simulink library "CoCoSTLib_R2015b"  (R2015b)
settings: Solver=ode45  StartTime=0.0  StopTime=10.0  RelTol=1e-3
libraries: CoCoSTLib_R2015b x31
settings Model: Creator=balsi  LastModifiedBy=xiayu
settings DataIOCC: SaveFormat=Array
settings DebuggingCC: AllowSymbolicDim=on
settings HardwareCC: ProdBitPerPointer=32  ProdLargestAtomicFloat=None  ProdIntDivRoundTo=Undefined  ProdEndianess=Unspecified  ProdWordSize=32  ProdHWDeviceType=32-bit Generic
settings ConfigComp: CovHtmlReporting=off  CovModelRefEnable=Off

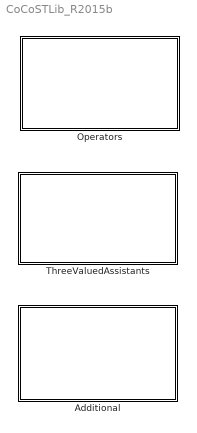
== system CoCoSTLib_R2015b ==
  Additional : Subsystem
      mask Display: disp('Additional')
  Operators : Subsystem
      mask Display: disp("Operators")
  ThreeValuedAssistants : Subsystem
      mask Display: disp("Enablers - Three Valued")

== system CoCoSTLib_R2015b/Additional ==
  note: Additional
  And_nested : Subsystem
  DelaySTL : Subsystem
  DelayedTimeWindow : Subsystem
  TimeWindow : Subsystem

== system CoCoSTLib_R2015b/Operators ==
  Operators_3V : Subsystem
      mask Display: disp("Operators Three-valued Logic")
  Operators_LF : Subsystem
      mask Display: disp('Operators LogicT')
  Operators_LT : Subsystem
      mask Display: disp('Operators LogicF')

== system CoCoSTLib_R2015b/ThreeValuedAssistants ==
  note: In order to save memory, values can be encoded in two digits.
      | For example:
      | 	True: [1, 1]
      |        False: [ 0, 0]
      |        Unknown: [1, 0]
  note: 3V assistants
  note: 3V assignments
  AND_3V : Subsystem
  False_3V : Subsystem
      mask Display: disp("F_3V")
  "Interpreter " : Subsystem
  NOT_3V : Subsystem
  OR_3V : Subsystem
  True_3V : Subsystem
      mask Display: disp("T_3V")
  Unknown_3V : Subsystem
      mask Display: disp("U_3V")

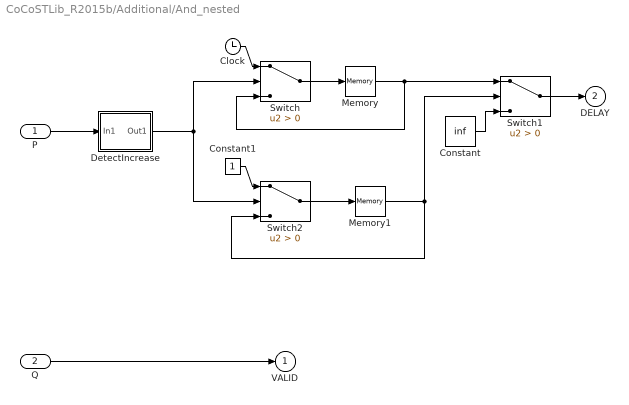
== system CoCoSTLib_R2015b/Additional/And_nested ==
  P : Inport
  Q : Inport  Port=2
  Clock : Clock
  Constant : Constant  Value=inf
  Constant1 : Constant
  DetectIncrease : Subsystem
  Memory : Memory
  Memory1 : Memory
  Switch : Switch  Criteria=u2 > Threshold
  Switch1 : Switch  Criteria=u2 > Threshold
  Switch2 : Switch  Criteria=u2 > Threshold
  VALID : Outport
  DELAY : Outport  Port=2
  wires:
  Q/1 -> VALID/1
  Memory/1 -> Switch1/1, Switch/3
  Memory1/1 -> Switch1/2, Switch2/3
  Switch/1 -> Memory/1
  Switch1/1 -> DELAY/1
  Constant/1 -> Switch1/3
  Switch2/1 -> Memory1/1
  Constant1/1 -> Switch2/1
  Clock/1 -> Switch/1
  DetectIncrease/1(Out1) -> Switch2/2, Switch/2
  P/1 -> DetectIncrease/1(In1)

== system CoCoSTLib_R2015b/Additional/DelaySTL ==
  IN : Inport
  Clock : Clock
  Constant : Constant  Value=inf
  Constant1 : Constant
  DetectIncrease : Subsystem
  Memory : Memory
  Memory1 : Memory
  Switch : Switch  Criteria=u2 > Threshold
  Switch1 : Switch  Criteria=u2 > Threshold
  Switch2 : Switch  Criteria=u2 > Threshold
  OUT : Outport
  wires:
  Clock/1 -> Switch/1
  Constant1/1 -> Switch2/1
  Memory1/1 -> Switch1/2, Switch2/3
  Switch/1 -> Memory/1
  Switch1/1 -> OUT/1
  Switch2/1 -> Memory1/1
  DetectIncrease/1(Y) -> Switch/2, Switch2/2
  IN/1 -> DetectIncrease/1(U)
  Memory/1 -> Switch1/1, Switch/3
  Constant/1 -> Switch1/3

== system CoCoSTLib_R2015b/Additional/DelayedTimeWindow ==
  T_Start : Inport
  T_End : Inport  Port=2
  DELAY : Inport  Port=3
  AND1 : Logic  AllPortsSameDT=off  OutDataTypeStr=boolean
  CLOCK : Clock
  DELAY_SUB : Sum  Inputs=+-
  REL1 : RelationalOperator  Operator=<=  OutDataTypeStr=boolean
  REL2 : RelationalOperator  Operator=<=  OutDataTypeStr=boolean
  OUT : Outport
  wires:
  REL1/1 -> AND1/1
  CLOCK/1 -> DELAY_SUB/1
  REL2/1 -> AND1/2
  T_Start/1 -> REL1/1
  DELAY_SUB/1 -> REL1/2, REL2/1
  AND1/1 -> OUT/1
  DELAY/1 -> DELAY_SUB/2
  T_End/1 -> REL2/2

== system CoCoSTLib_R2015b/Additional/TimeWindow ==
  T_Start : Inport
  T_End : Inport  Port=2
  AND : Logic  AllPortsSameDT=off  OutDataTypeStr=boolean
  CLOCK : Clock
  REL1 : RelationalOperator  Operator=<=  OutDataTypeStr=boolean
  REL2 : RelationalOperator  Operator=<=  OutDataTypeStr=boolean
  OUT : Outport
  wires:
  CLOCK/1 -> REL1/2, REL2/1
  T_End/1 -> REL2/2
  REL1/1 -> AND/1
  REL2/1 -> AND/2
  AND/1 -> OUT/1
  T_Start/1 -> REL1/1

== system CoCoSTLib_R2015b/Operators/Operators_3V ==
  Always_3V : Subsystem
  Eventually_3V : Subsystem
  Until_3V : Subsystem

== system CoCoSTLib_R2015b/Operators/Operators_LF ==
  Always_LF : Subsystem
  Eventually_LF : Subsystem
      mask Display: disp('Eventuall LogicF')
  Eventually_LFbis : Subsystem  Commented=on
  Until_LF : Subsystem

== system CoCoSTLib_R2015b/Operators/Operators_LT ==
  "Always_LT " : Subsystem
  Always_LT_timewindows : Subsystem  Commented=on
  Always_LTbis : Subsystem  Commented=on
  "Eventually_LT " : Subsystem
  Eventually_LT bis : Subsystem  Commented=on
  Eventually_T : Subsystem  Commented=on
  Until_LT : Subsystem

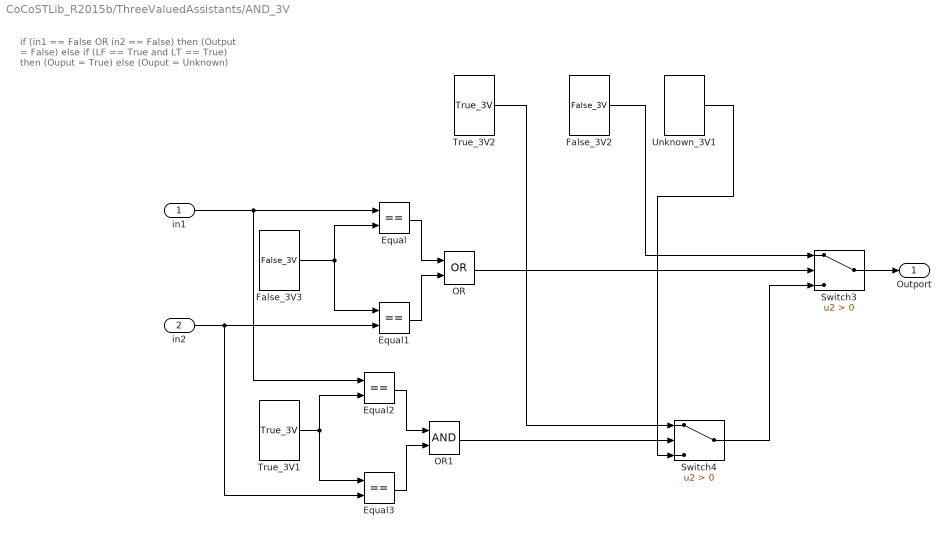
== system CoCoSTLib_R2015b/ThreeValuedAssistants/AND_3V ==
  note: if (in1 == False OR in2 == False)
      | then (Output = False)
      | else if (LF == True and LT == True)
      | then (Ouput = True)
      | else (Ouput = Unknown)
  "in1 " : Inport
  in2 : Inport  Port=2
  Equal{,1..3} (4 alike) : RelationalOperator  Operator===  OutDataTypeStr=boolean
  False_3V2 : CoCoSTLib_R2015b/ThreeValuedAssistants/False_3V  SystemSampleTime=-1  Latency=0  AutoFrameSizeCalculation=off
  False_3V3 : CoCoSTLib_R2015b/ThreeValuedAssistants/False_3V  SystemSampleTime=-1  Latency=0  AutoFrameSizeCalculation=off
  OR : Logic  Operator=OR  AllPortsSameDT=off  OutDataTypeStr=boolean
  OR1 : Logic  AllPortsSameDT=off  OutDataTypeStr=boolean
  Switch3 : Switch  Criteria=u2 > Threshold
  Switch4 : Switch  Criteria=u2 > Threshold
  True_3V1 : CoCoSTLib_R2015b/ThreeValuedAssistants/True_3V  SystemSampleTime=-1  Latency=0  AutoFrameSizeCalculation=off
  True_3V2 : CoCoSTLib_R2015b/ThreeValuedAssistants/True_3V  SystemSampleTime=-1  Latency=0  AutoFrameSizeCalculation=off
  Unknown_3V1 : CoCoSTLib_R2015b/ThreeValuedAssistants/Unknown_3V  SystemSampleTime=-1  Latency=0  AutoFrameSizeCalculation=off
  Outport : Outport
  wires:
  False_3V3/1 -> Equal/2, Equal1/1
  Equal/1 -> OR/1
  Equal1/1 -> OR/2
  OR/1 -> Switch3/2
  Switch3/1 -> Outport/1
  Equal2/1 -> OR1/1
  Equal3/1 -> OR1/2
  OR1/1 -> Switch4/2
  "in1 "/1 -> Equal2/1, Equal/1
  True_3V1/1 -> Equal2/2, Equal3/1
  in2/1 -> Equal1/2, Equal3/2
  True_3V2/1 -> Switch4/1
  Switch4/1 -> Switch3/3
  False_3V2/1 -> Switch3/1
  Unknown_3V1/1 -> Switch4/3

== system CoCoSTLib_R2015b/ThreeValuedAssistants/False_3V ==
  Constant1 : Constant  Value=0
  Out1 : Outport
  wires:
  Constant1/1 -> Out1/1

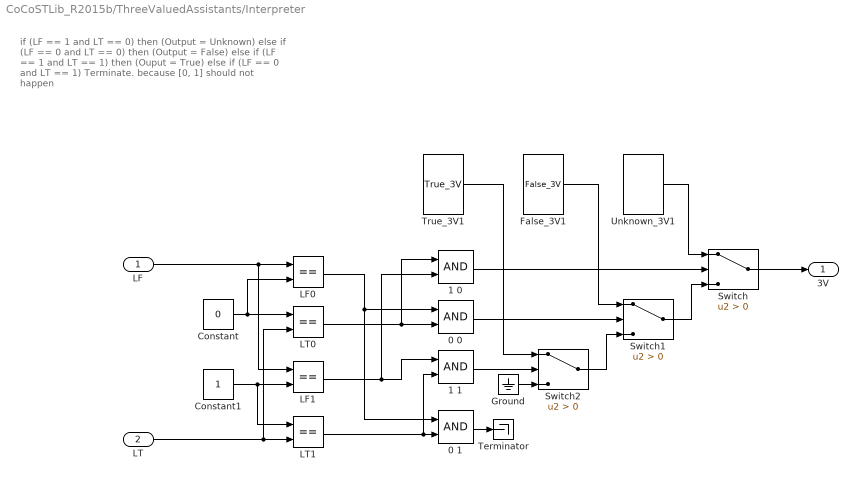
== system CoCoSTLib_R2015b/ThreeValuedAssistants/Interpreter  ==
  note: if (LF == 1 and LT == 0)
      | then (Output = Unknown)
      | else if (LF == 0 and LT == 0)
      | then (Output = False)
      | else if (LF == 1 and LT == 1)
      | then (Ouput = True)
      | else if (LF == 0 and LT == 1)
      | Terminate.
      | because [0, 1] should not happen
  LF : Inport
  LT : Inport  Port=2
  0 0 : Logic  AllPortsSameDT=off  OutDataTypeStr=boolean
  0 1 : Logic  AllPortsSameDT=off  OutDataTypeStr=boolean
  1 0 : Logic  AllPortsSameDT=off  OutDataTypeStr=boolean
  1 1 : Logic  AllPortsSameDT=off  OutDataTypeStr=boolean
  Constant : Constant  Value=0
  Constant1 : Constant
  False_3V1 : CoCoSTLib_R2015b/ThreeValuedAssistants/False_3V  SystemSampleTime=-1  Latency=0  AutoFrameSizeCalculation=off
  Ground : Ground
  LF0 : RelationalOperator  Operator===  OutDataTypeStr=boolean
  LF1 : RelationalOperator  Operator===  OutDataTypeStr=boolean
  "LT0 " : RelationalOperator  Operator===  OutDataTypeStr=boolean
  "LT1 " : RelationalOperator  Operator===  OutDataTypeStr=boolean
  Switch : Switch  Criteria=u2 > Threshold
  Switch1 : Switch  Criteria=u2 > Threshold
  Switch2 : Switch  Criteria=u2 > Threshold
  Terminator : Terminator
  True_3V1 : CoCoSTLib_R2015b/ThreeValuedAssistants/True_3V  SystemSampleTime=-1  Latency=0  AutoFrameSizeCalculation=off
  Unknown_3V1 : CoCoSTLib_R2015b/ThreeValuedAssistants/Unknown_3V  SystemSampleTime=-1  Latency=0  AutoFrameSizeCalculation=off
  3V : Outport
  wires:
  Constant/1 -> "LT0 "/1, LF0/2
  1 0/1 -> Switch/2
  Switch/1 -> 3V/1
  Constant1/1 -> LF1/2, "LT1 "/1
  LF1/1 -> 1 1/1, 1 0/2
  0 0/1 -> Switch1/2
  Switch1/1 -> Switch/3
  "LT0 "/1 -> 0 0/2, 1 0/1
  LF0/1 -> 0 1/1, 0 0/1
  "LT1 "/1 -> 1 1/2, 0 1/2
  1 1/1 -> Switch2/2
  Switch2/1 -> Switch1/3
  0 1/1 -> Terminator/1
  Ground/1 -> Switch2/3
  Unknown_3V1/1 -> Switch/1
  True_3V1/1 -> Switch2/1
  False_3V1/1 -> Switch1/1
  LF/1 -> LF1/1, LF0/1
  LT/1 -> "LT0 "/2, "LT1 "/2

== system CoCoSTLib_R2015b/ThreeValuedAssistants/NOT_3V ==
  note: if (in == True)
      | then (Output = False)
      | else if (in == False)
      | then (Ouput = True)
      | else (Ouput = Unknown)
  "Input " : Inport
  Equal : RelationalOperator  Operator===  OutDataTypeStr=boolean
  Equal2 : RelationalOperator  Operator===  OutDataTypeStr=boolean
  False_3V1 : CoCoSTLib_R2015b/ThreeValuedAssistants/False_3V  SystemSampleTime=-1  Latency=0  AutoFrameSizeCalculation=off
  False_3V2 : CoCoSTLib_R2015b/ThreeValuedAssistants/False_3V  SystemSampleTime=-1  Latency=0  AutoFrameSizeCalculation=off
  Switch3 : Switch  Criteria=u2 > Threshold
  Switch4 : Switch  Criteria=u2 > Threshold
  True_3V2 : CoCoSTLib_R2015b/ThreeValuedAssistants/True_3V  SystemSampleTime=-1  Latency=0  AutoFrameSizeCalculation=off
  True_3V3 : CoCoSTLib_R2015b/ThreeValuedAssistants/True_3V  SystemSampleTime=-1  Latency=0  AutoFrameSizeCalculation=off
  Unknown_3V1 : CoCoSTLib_R2015b/ThreeValuedAssistants/Unknown_3V  SystemSampleTime=-1  Latency=0  AutoFrameSizeCalculation=off
  Outport : Outport
  wires:
  Switch3/1 -> Outport/1
  False_3V1/1 -> Equal2/2
  Equal/1 -> Switch3/2
  "Input "/1 -> Equal2/1, Equal/1
  False_3V2/1 -> Switch3/1
  True_3V3/1 -> Equal/2
  Unknown_3V1/1 -> Switch4/3
  Switch4/1 -> Switch3/3
  True_3V2/1 -> Switch4/1
  Equal2/1 -> Switch4/2

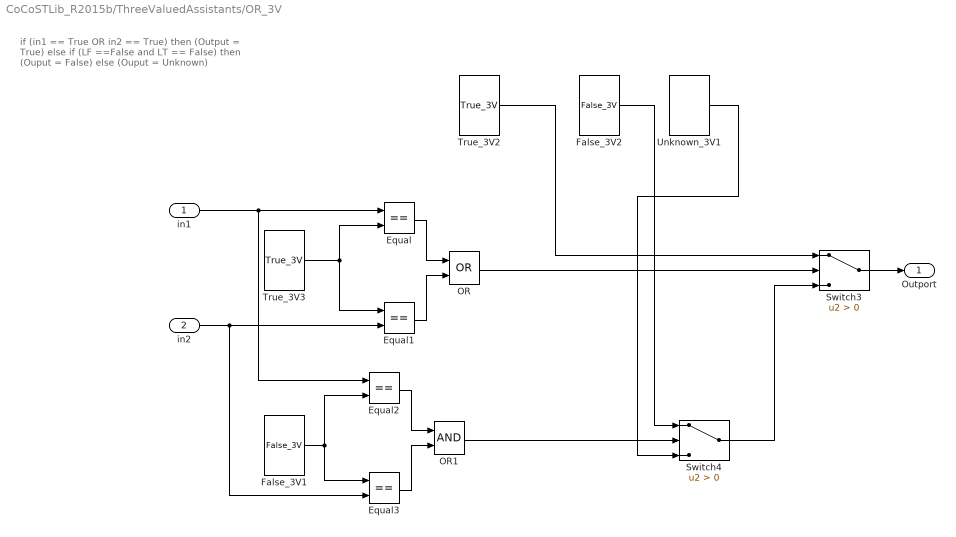
== system CoCoSTLib_R2015b/ThreeValuedAssistants/OR_3V ==
  note: if (in1 == True OR in2 == True)
      | then (Output = True)
      | else if (LF ==False and LT == False)
      | then (Ouput = False)
      | else (Ouput = Unknown)
  "in1 " : Inport
  in2 : Inport  Port=2
  Equal{,1..3} (4 alike) : RelationalOperator  Operator===  OutDataTypeStr=boolean
  False_3V1 : CoCoSTLib_R2015b/ThreeValuedAssistants/False_3V  SystemSampleTime=-1  Latency=0  AutoFrameSizeCalculation=off
  False_3V2 : CoCoSTLib_R2015b/ThreeValuedAssistants/False_3V  SystemSampleTime=-1  Latency=0  AutoFrameSizeCalculation=off
  OR : Logic  Operator=OR  AllPortsSameDT=off  OutDataTypeStr=boolean
  OR1 : Logic  AllPortsSameDT=off  OutDataTypeStr=boolean
  Switch3 : Switch  Criteria=u2 > Threshold
  Switch4 : Switch  Criteria=u2 > Threshold
  True_3V2 : CoCoSTLib_R2015b/ThreeValuedAssistants/True_3V  SystemSampleTime=-1  Latency=0  AutoFrameSizeCalculation=off
  True_3V3 : CoCoSTLib_R2015b/ThreeValuedAssistants/True_3V  SystemSampleTime=-1  Latency=0  AutoFrameSizeCalculation=off
  Unknown_3V1 : CoCoSTLib_R2015b/ThreeValuedAssistants/Unknown_3V  SystemSampleTime=-1  Latency=0  AutoFrameSizeCalculation=off
  Outport : Outport
  wires:
  True_3V3/1 -> Equal/2, Equal1/1
  Equal/1 -> OR/1
  Equal1/1 -> OR/2
  OR/1 -> Switch3/2
  Unknown_3V1/1 -> Switch4/3
  Switch3/1 -> Outport/1
  Equal2/1 -> OR1/1
  Equal3/1 -> OR1/2
  OR1/1 -> Switch4/2
  "in1 "/1 -> Equal2/1, Equal/1
  False_3V1/1 -> Equal2/2, Equal3/1
  in2/1 -> Equal1/2, Equal3/2
  False_3V2/1 -> Switch4/1
  Switch4/1 -> Switch3/3
  True_3V2/1 -> Switch3/1

== system CoCoSTLib_R2015b/ThreeValuedAssistants/True_3V ==
  Constant : Constant
  Out1 : Outport
  wires:
  Constant/1 -> Out1/1

== system CoCoSTLib_R2015b/ThreeValuedAssistants/Unknown_3V ==
  Constant2 : Constant  Value=-1
  Out1 : Outport
  wires:
  Constant2/1 -> Out1/1

== system CoCoSTLib_R2015b/Additional/And_nested/DetectIncrease ==
  note: U(k)
  note: Edge
  In1 : Inport
  FixPt Relational Operator : RelationalOperator  Operator=>  OutDataTypeStr=boolean  ZeroCross=off
  Memory : Memory
  Out1 : Outport
  wires:
  In1/1 -> Memory/1, FixPt Relational Operator/1
  Memory/1 -> FixPt Relational Operator/2  "U(k-1)"
  FixPt Relational Operator/1 -> Out1/1

== system CoCoSTLib_R2015b/Additional/DelaySTL/DetectIncrease ==
  note: U(k)
  note: Edge
  U : Inport
  FixPt Relational Operator : RelationalOperator  Operator=>  OutDataTypeStr=boolean  ZeroCross=off
  Memory : Memory
  Y : Outport  InitialOutput=0
  wires:
  Memory/1 -> FixPt Relational Operator/2  "U(k-1)"
  FixPt Relational Operator/1 -> Y/1
  U/1 -> Memory/1, FixPt Relational Operator/1

== system CoCoSTLib_R2015b/Operators/Operators_3V/Always_3V ==
  "T_start " : Inport
  "T_end " : Inport  Port=2
  P : Inport  Port=3
  Always LF : CoCoSTLib_R2015b/Operators/Operators_LF/Always_LF  SystemSampleTime=-1  Latency=0  AutoFrameSizeCalculation=off
  "Always LT " : CoCoSTLib_R2015b/Operators/Operators_LT/Always_LT   SystemSampleTime=-1  Latency=0  AutoFrameSizeCalculation=off
  "Interpreter " : CoCoSTLib_R2015b/ThreeValuedAssistants/Interpreter   SystemSampleTime=-1  Latency=0  AutoFrameSizeCalculation=off
  3V : Outport
  wires:
  "T_end "/1 -> "Always LT "/2, Always LF/2
  Always LF/1 -> "Interpreter "/1
  "Interpreter "/1 -> 3V/1
  "T_start "/1 -> Always LF/1, "Always LT "/1
  P/1 -> Always LF/3, "Always LT "/3
  "Always LT "/1 -> "Interpreter "/2

== system CoCoSTLib_R2015b/Operators/Operators_3V/Eventually_3V ==
  "T_start " : Inport
  "T_end " : Inport  Port=2
  P : Inport  Port=3
  Eventually LF : CoCoSTLib_R2015b/Operators/Operators_LF/Eventually_LF  SystemSampleTime=-1  Latency=0  AutoFrameSizeCalculation=off
  "Eventually LT " : CoCoSTLib_R2015b/Operators/Operators_LT/Eventually_LT   SystemSampleTime=-1  Latency=0  AutoFrameSizeCalculation=off
  "Interpreter " : CoCoSTLib_R2015b/ThreeValuedAssistants/Interpreter   SystemSampleTime=-1  Latency=0  AutoFrameSizeCalculation=off
  3V : Outport
  wires:
  Eventually LF/1 -> "Interpreter "/1
  "Eventually LT "/1 -> "Interpreter "/2
  P/1 -> "Eventually LT "/3, Eventually LF/3
  "T_end "/1 -> "Eventually LT "/2, Eventually LF/2
  "Interpreter "/1 -> 3V/1
  "T_start "/1 -> "Eventually LT "/1, Eventually LF/1

== system CoCoSTLib_R2015b/Operators/Operators_3V/Until_3V ==
  "T_start " : Inport
  "T_end " : Inport  Port=2
  P : Inport  Port=3
  "Q " : Inport  Port=4
  "Interpreter " : CoCoSTLib_R2015b/ThreeValuedAssistants/Interpreter   SystemSampleTime=-1  Latency=0  AutoFrameSizeCalculation=off
  Until LF : CoCoSTLib_R2015b/Operators/Operators_LF/Until_LF  SystemSampleTime=-1  Latency=0  AutoFrameSizeCalculation=off
  Until LT : CoCoSTLib_R2015b/Operators/Operators_LT/Until_LT  SystemSampleTime=-1  Latency=0  AutoFrameSizeCalculation=off
  3V : Outport
  wires:
  "T_end "/1 -> Until LF/2, Until LT/2
  "T_start "/1 -> Until LT/1, Until LF/1
  "Q "/1 -> Until LF/4, Until LT/4
  P/1 -> Until LF/3, Until LT/3
  "Interpreter "/1 -> 3V/1
  Until LT/1 -> "Interpreter "/2
  Until LF/1 -> "Interpreter "/1

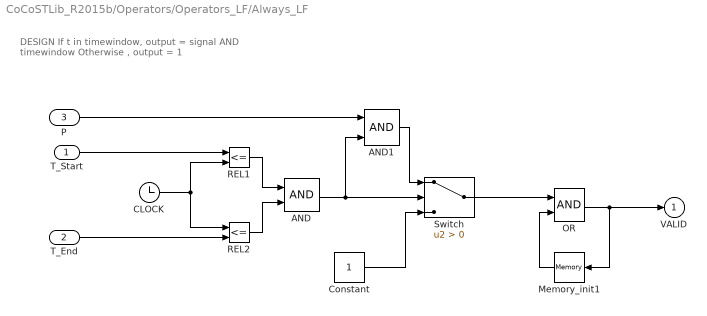
== system CoCoSTLib_R2015b/Operators/Operators_LF/Always_LF ==
  note: DESIGN
      | If t in timewindow, output = signal AND timewindow
      | Otherwise , output = 1
  T_Start : Inport
  T_End : Inport  Port=2
  P : Inport  Port=3
  AND : Logic  AllPortsSameDT=off  OutDataTypeStr=boolean
  AND1 : Logic  AllPortsSameDT=off  OutDataTypeStr=boolean
  CLOCK : Clock
  Constant : Constant
  Memory_init1 : Memory  X0=1
  OR : Logic  AllPortsSameDT=off  OutDataTypeStr=boolean
  REL1 : RelationalOperator  Operator=<=  OutDataTypeStr=boolean
  REL2 : RelationalOperator  Operator=<=  OutDataTypeStr=boolean
  Switch : Switch  Criteria=u2 > Threshold
  VALID : Outport
  wires:
  AND1/1 -> Switch/1
  CLOCK/1 -> REL2/1, REL1/2
  Memory_init1/1 -> OR/2
  Switch/1 -> OR/1
  T_End/1 -> REL2/2
  OR/1 -> VALID/1, Memory_init1/1
  T_Start/1 -> REL1/1
  Constant/1 -> Switch/3
  REL1/1 -> AND/1
  REL2/1 -> AND/2
  AND/1 -> AND1/2, Switch/2
  P/1 -> AND1/1

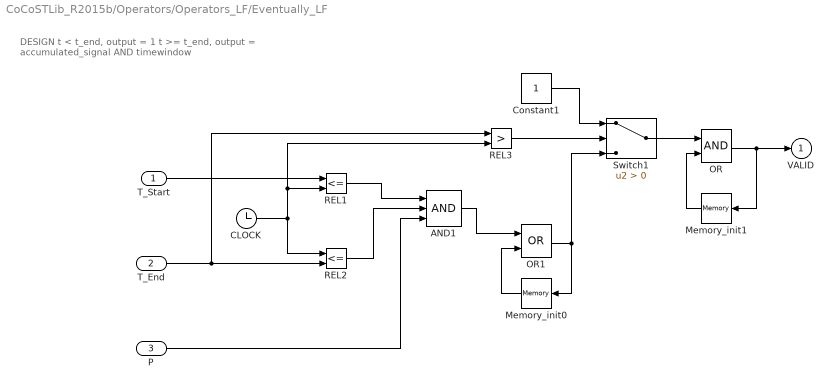
== system CoCoSTLib_R2015b/Operators/Operators_LF/Eventually_LF ==
  note: DESIGN
      | t < t_end, output = 1
      | t >= t_end, output = accumulated_signal AND timewindow
  T_Start : Inport
  T_End : Inport  Port=2
  P : Inport  Port=3
  AND1 : Logic  Inputs=3  AllPortsSameDT=off  OutDataTypeStr=boolean
  CLOCK : Clock
  Constant1 : Constant
  "Memory_init0 " : Memory
  Memory_init1 : Memory  X0=1
  OR : Logic  AllPortsSameDT=off  OutDataTypeStr=boolean
  OR1 : Logic  Operator=OR  AllPortsSameDT=off  OutDataTypeStr=boolean
  REL1 : RelationalOperator  Operator=<=  OutDataTypeStr=boolean
  REL2 : RelationalOperator  Operator=<=  OutDataTypeStr=boolean
  REL3 : RelationalOperator  Operator=>  OutDataTypeStr=boolean
  Switch1 : Switch  Criteria=u2 > Threshold
  VALID : Outport
  wires:
  T_End/1 -> REL3/1, REL2/2
  AND1/1 -> OR1/1
  REL1/1 -> AND1/1
  P/1 -> AND1/3
  CLOCK/1 -> REL3/2, REL1/2, REL2/1
  T_Start/1 -> REL1/1
  "Memory_init0 "/1 -> OR1/2
  OR1/1 -> "Memory_init0 "/1, Switch1/3
  Constant1/1 -> Switch1/1
  REL2/1 -> AND1/2
  REL3/1 -> Switch1/2
  Memory_init1/1 -> OR/2
  OR/1 -> VALID/1, Memory_init1/1
  Switch1/1 -> OR/1

== system CoCoSTLib_R2015b/Operators/Operators_LF/Eventually_LFbis ==
  note: DESIGN
      | t < t_end, output = 1
      | t >= t_end, output = accumulated_signal AND timewindow
  T_Start : Inport
  T_End : Inport  Port=2
  P : Inport  Port=3
  AND2 : Logic  AllPortsSameDT=off  OutDataTypeStr=boolean
  Always LF : CoCoSTLib_R2015b/Operators_LF/Always_LF  SystemSampleTime=-1  Latency=0  AutoFrameSizeCalculation=off
  CLOCK1 : Clock
  Memory_init1 : Memory  X0=1
  NOT : Logic  Operator=NOT  IconShape=distinctive  AllPortsSameDT=off  OutDataTypeStr=boolean
  NOT1 : Logic  Operator=NOT  IconShape=distinctive  AllPortsSameDT=off  OutDataTypeStr=boolean
  OR : Logic  AllPortsSameDT=off  OutDataTypeStr=boolean
  REL4 : RelationalOperator  Operator=<=  OutDataTypeStr=boolean
  VALID : Outport
  wires:
  T_Start/1 -> Always LF/1
  T_End/1 -> Always LF/2, REL4/1
  P/1 -> NOT/1
  NOT/1 -> Always LF/3
  CLOCK1/1 -> REL4/2
  Always LF/1 -> AND2/1
  REL4/1 -> AND2/2
  AND2/1 -> NOT1/1
  Memory_init1/1 -> OR/2
  NOT1/1 -> OR/1
  OR/1 -> VALID/1, Memory_init1/1

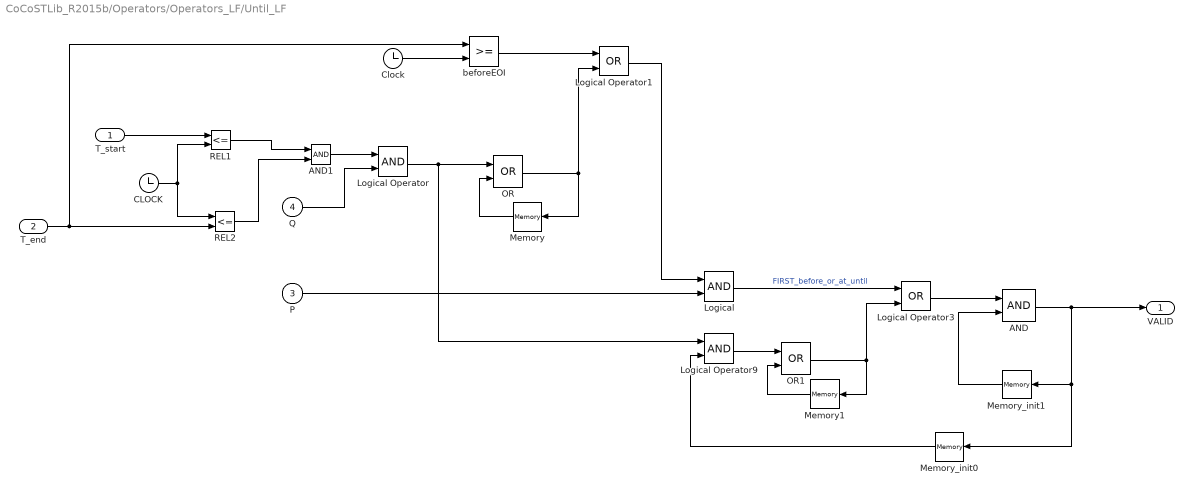
== system CoCoSTLib_R2015b/Operators/Operators_LF/Until_LF ==
  "T_start " : Inport
  T_end : Inport  Port=2
  P : Inport  Port=3
  Q : Inport  Port=4
  AND : Logic  AllPortsSameDT=off  OutDataTypeStr=boolean
  AND1 : Logic  AllPortsSameDT=off  OutDataTypeStr=boolean
  CLOCK : Clock
  Clock : Clock
  "Logical " : Logic  AllPortsSameDT=off  OutDataTypeStr=boolean
  Logical Operator : Logic  AllPortsSameDT=off  OutDataTypeStr=boolean
  Logical Operator1 : Logic  Operator=OR  AllPortsSameDT=off  OutDataTypeStr=boolean
  Logical Operator3 : Logic  Operator=OR  AllPortsSameDT=off  OutDataTypeStr=boolean
  Logical Operator9 : Logic  AllPortsSameDT=off  OutDataTypeStr=boolean
  Memory : Memory
  Memory1 : Memory
  "Memory_init0 " : Memory
  Memory_init1 : Memory  X0=1
  OR : Logic  Operator=OR  AllPortsSameDT=off  OutDataTypeStr=boolean
  OR1 : Logic  Operator=OR  AllPortsSameDT=off  OutDataTypeStr=boolean
  REL1 : RelationalOperator  Operator=<=  OutDataTypeStr=boolean
  REL2 : RelationalOperator  Operator=<=  OutDataTypeStr=boolean
  beforeEOI : RelationalOperator  OutDataTypeStr=boolean
  VALID : Outport
  wires:
  Memory1/1 -> OR1/2
  Logical Operator1/1 -> "Logical "/1
  beforeEOI/1 -> Logical Operator1/1
  REL2/1 -> AND1/2
  P/1 -> "Logical "/2
  AND1/1 -> Logical Operator/1
  Logical Operator3/1 -> AND/1
  REL1/1 -> AND1/1
  OR/1 -> Memory/1, Logical Operator1/2
  "Logical "/1 -> Logical Operator3/1  "FIRST_before_or_at_until"
  "T_start "/1 -> REL1/1
  Logical Operator9/1 -> OR1/1
  AND/1 -> VALID/1, "Memory_init0 "/1, Memory_init1/1
  Logical Operator/1 -> OR/1, Logical Operator9/1
  Memory/1 -> OR/2
  CLOCK/1 -> REL2/1, REL1/2
  Q/1 -> Logical Operator/2
  "Memory_init0 "/1 -> Logical Operator9/2
  T_end/1 -> beforeEOI/1, REL2/2
  OR1/1 -> Memory1/1, Logical Operator3/2
  Memory_init1/1 -> AND/2
  Clock/1 -> beforeEOI/2

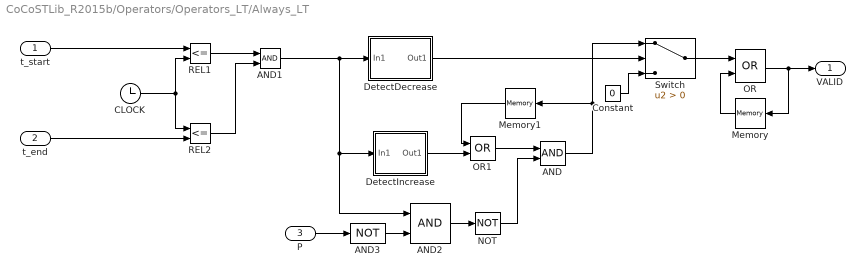
== system CoCoSTLib_R2015b/Operators/Operators_LT/Always_LT  ==
  t_start : Inport
  t_end : Inport  Port=2
  P : Inport  Port=3
  AND : Logic  AllPortsSameDT=off  OutDataTypeStr=boolean
  AND1 : Logic  AllPortsSameDT=off  OutDataTypeStr=boolean
  AND2 : Logic  AllPortsSameDT=off  OutDataTypeStr=boolean
  AND3 : Logic  Operator=NOT  AllPortsSameDT=off  OutDataTypeStr=boolean
  CLOCK : Clock
  Constant : Constant  Value=0  OutDataTypeStr=boolean
  "DetectDecrease " : Subsystem
  DetectIncrease : Subsystem
  Memory : Memory
  Memory1 : Memory
  NOT : Logic  Operator=NOT  AllPortsSameDT=off  OutDataTypeStr=boolean
  OR : Logic  Operator=OR  AllPortsSameDT=off  OutDataTypeStr=boolean
  OR1 : Logic  Operator=OR  AllPortsSameDT=off  OutDataTypeStr=boolean
  REL1 : RelationalOperator  Operator=<=  OutDataTypeStr=boolean
  REL2 : RelationalOperator  Operator=<=  OutDataTypeStr=boolean
  Switch : Switch  Criteria=u2 > Threshold
  VALID : Outport
  wires:
  OR/1 -> Memory/1, VALID/1
  NOT/1 -> AND/2
  AND3/1 -> AND2/2
  Memory/1 -> OR/2
  AND/1 -> Memory1/1, Switch/1
  OR1/1 -> AND/1
  P/1 -> AND3/1
  Memory1/1 -> OR1/1
  AND2/1 -> NOT/1
  Switch/1 -> OR/1
  Constant/1 -> Switch/3
  t_end/1 -> REL2/2
  CLOCK/1 -> REL1/2, REL2/1
  REL2/1 -> AND1/2
  REL1/1 -> AND1/1
  t_start/1 -> REL1/1
  "DetectDecrease "/1(Out1) -> Switch/2
  AND1/1 -> AND2/1, DetectIncrease/1(In1), "DetectDecrease "/1(In1)
  DetectIncrease/1(Out1) -> OR1/2

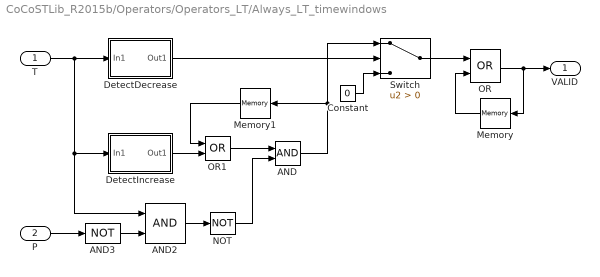
== system CoCoSTLib_R2015b/Operators/Operators_LT/Always_LT_timewindows ==
  T : Inport
  P : Inport  Port=2
  AND : Logic  AllPortsSameDT=off  OutDataTypeStr=boolean
  AND2 : Logic  AllPortsSameDT=off  OutDataTypeStr=boolean
  AND3 : Logic  Operator=NOT  AllPortsSameDT=off  OutDataTypeStr=boolean
  Constant : Constant  Value=0  OutDataTypeStr=boolean
  DetectDecrease : Subsystem
  DetectIncrease : Subsystem
  Memory : Memory
  Memory1 : Memory
  NOT : Logic  Operator=NOT  AllPortsSameDT=off  OutDataTypeStr=boolean
  OR : Logic  Operator=OR  AllPortsSameDT=off  OutDataTypeStr=boolean
  OR1 : Logic  Operator=OR  AllPortsSameDT=off  OutDataTypeStr=boolean
  Switch : Switch  Criteria=u2 > Threshold
  VALID : Outport
  wires:
  AND2/1 -> NOT/1
  DetectIncrease/1(Out1) -> OR1/2
  DetectDecrease/1(Out1) -> Switch/2
  AND/1 -> Memory1/1, Switch/1
  AND3/1 -> AND2/2
  T/1 -> AND2/1, DetectIncrease/1(In1), DetectDecrease/1(In1)
  P/1 -> AND3/1
  Constant/1 -> Switch/3
  Switch/1 -> OR/1
  OR/1 -> Memory/1, VALID/1
  Memory/1 -> OR/2
  Memory1/1 -> OR1/1
  OR1/1 -> AND/1
  NOT/1 -> AND/2

== system CoCoSTLib_R2015b/Operators/Operators_LT/Always_LTbis ==
  T_Start : Inport
  T_End : Inport  Port=2
  P : Inport  Port=3
  AND2 : Logic  Inputs=3  AllPortsSameDT=off  OutDataTypeStr=boolean
  CLOCK : Clock
  Memory : Memory
  NOT : Logic  Operator=NOT  IconShape=distinctive  AllPortsSameDT=off  OutDataTypeStr=boolean
  NOT1 : Logic  Operator=NOT  IconShape=distinctive  AllPortsSameDT=off  OutDataTypeStr=boolean
  OR : Logic  Operator=OR  AllPortsSameDT=off  OutDataTypeStr=boolean
  REL1 : RelationalOperator  Operator=<=  OutDataTypeStr=boolean
  REL2 : RelationalOperator  Operator=<=  OutDataTypeStr=boolean
  VALID : Outport
  wires:
  AND2/1 -> NOT/1
  P/1 -> NOT1/1
  REL1/1 -> AND2/2
  REL2/1 -> AND2/3
  T_Start/1 -> REL1/1
  T_End/1 -> REL2/2
  CLOCK/1 -> REL2/1, REL1/2
  Memory/1 -> OR/2
  OR/1 -> VALID/1, Memory/1
  NOT1/1 -> AND2/1
  NOT/1 -> OR/1

== system CoCoSTLib_R2015b/Operators/Operators_LT/Eventually_LT  ==
  T_Start : Inport
  T_End : Inport  Port=2
  P : Inport  Port=3
  AND2 : Logic  Inputs=3  AllPortsSameDT=off  OutDataTypeStr=boolean
  CLOCK : Clock
  Memory : Memory
  OR : Logic  Operator=OR  AllPortsSameDT=off  OutDataTypeStr=boolean
  REL1 : RelationalOperator  Operator=<=  OutDataTypeStr=boolean
  REL2 : RelationalOperator  Operator=<=  OutDataTypeStr=boolean
  VALID : Outport
  wires:
  REL1/1 -> AND2/2
  T_Start/1 -> REL1/1
  P/1 -> AND2/1
  REL2/1 -> AND2/3
  T_End/1 -> REL2/2
  CLOCK/1 -> REL1/2, REL2/1
  OR/1 -> Memory/1, VALID/1
  AND2/1 -> OR/1
  Memory/1 -> OR/2

== system CoCoSTLib_R2015b/Operators/Operators_LT/Eventually_LT bis ==
  T_Start : Inport
  T_End : Inport  Port=2
  P : Inport  Port=3
  AND2 : Logic  Inputs=3  AllPortsSameDT=off  OutDataTypeStr=boolean
  CLOCK : Clock
  Memory : Memory
  OR : Logic  Operator=OR  AllPortsSameDT=off  OutDataTypeStr=boolean
  REL1 : RelationalOperator  Operator=<=  OutDataTypeStr=boolean
  REL2 : RelationalOperator  Operator=<=  OutDataTypeStr=boolean
  VALID : Outport
  wires:
  Memory/1 -> OR/2
  AND2/1 -> OR/1
  OR/1 -> VALID/1, Memory/1
  CLOCK/1 -> REL2/1, REL1/2
  T_End/1 -> REL2/2
  REL2/1 -> AND2/3
  P/1 -> AND2/1
  T_Start/1 -> REL1/1
  REL1/1 -> AND2/2

== system CoCoSTLib_R2015b/Operators/Operators_LT/Eventually_T ==
  "T " : Inport
  P : Inport  Port=2
  AND2 : Logic  AllPortsSameDT=off  OutDataTypeStr=boolean
  Memory : Memory
  OR : Logic  Operator=OR  AllPortsSameDT=off  OutDataTypeStr=boolean
  VALID : Outport
  wires:
  AND2/1 -> OR/1
  OR/1 -> Memory/1, VALID/1
  "T "/1 -> AND2/2
  P/1 -> AND2/1
  Memory/1 -> OR/2

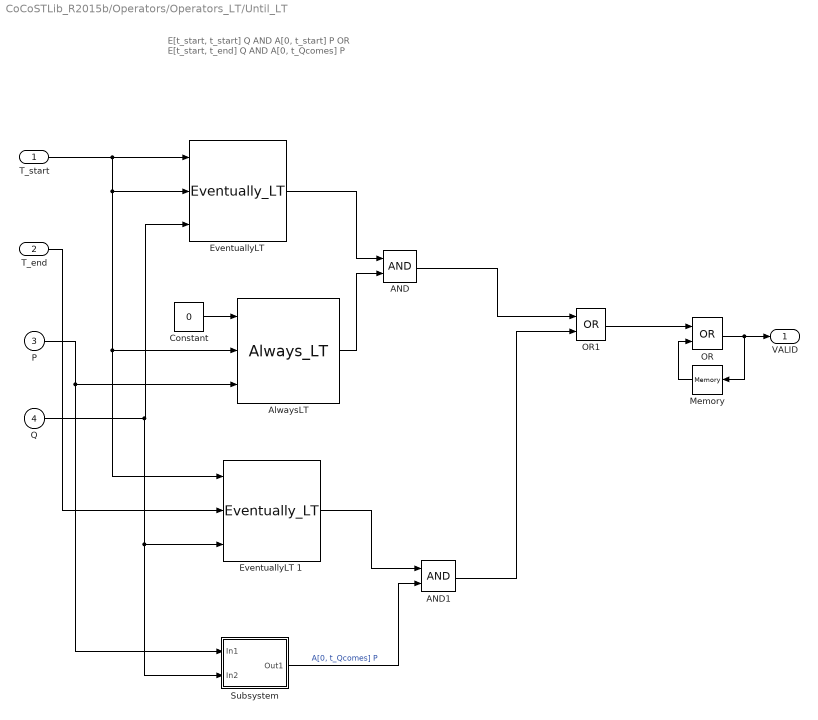
== system CoCoSTLib_R2015b/Operators/Operators_LT/Until_LT ==
  note: E[t_start, t_start] Q AND A[0, t_start] P
      | OR
      | E[t_start, t_end] Q AND A[0, t_Qcomes] P
  "T_start " : Inport
  T_end : Inport  Port=2
  P : Inport  Port=3
  Q : Inport  Port=4
  AND : Logic  AllPortsSameDT=off  OutDataTypeStr=boolean
  AND1 : Logic  AllPortsSameDT=off  OutDataTypeStr=boolean
  "AlwaysLT " : CoCoSTLib_R2015b/Operators/Operators_LT/Always_LT   SystemSampleTime=-1  Latency=0  AutoFrameSizeCalculation=off
  Constant : Constant  Value=0
  "EventuallyLT " : CoCoSTLib_R2015b/Operators/Operators_LT/Eventually_LT   SystemSampleTime=-1  Latency=0  AutoFrameSizeCalculation=off
  EventuallyLT 1 : CoCoSTLib_R2015b/Operators/Operators_LT/Eventually_LT   SystemSampleTime=-1  Latency=0  AutoFrameSizeCalculation=off
  Memory : Memory
  OR : Logic  Operator=OR  AllPortsSameDT=off  OutDataTypeStr=boolean
  OR1 : Logic  Operator=OR  AllPortsSameDT=off  OutDataTypeStr=boolean
  Subsystem : Subsystem
  VALID : Outport
  wires:
  "T_start "/1 -> EventuallyLT 1/1, "AlwaysLT "/2, "EventuallyLT "/2, "EventuallyLT "/1
  Constant/1 -> "AlwaysLT "/1
  "AlwaysLT "/1 -> AND/2
  "EventuallyLT "/1 -> AND/1
  OR/1 -> VALID/1, Memory/1
  Memory/1 -> OR/2
  OR1/1 -> OR/1
  AND/1 -> OR1/1
  T_end/1 -> EventuallyLT 1/2
  EventuallyLT 1/1 -> AND1/1
  AND1/1 -> OR1/2
  Q/1 -> Subsystem/2(In2), EventuallyLT 1/3, "EventuallyLT "/3
  P/1 -> Subsystem/1(In1), "AlwaysLT "/3
  Subsystem/1(Out1) -> AND1/2  "A[0, t_Qcomes] P"

== system CoCoSTLib_R2015b/Operators/Operators_LT/Always_LT /DetectDecrease  ==
  note: U(k)
  note: Edge
  In1 : Inport
  FixPt Relational Operator : RelationalOperator  Operator=<  OutDataTypeStr=boolean  ZeroCross=off
  Memory : Memory
  Out1 : Outport
  wires:
  FixPt Relational Operator/1 -> Out1/1
  Memory/1 -> FixPt Relational Operator/2  "U(k-1)"
  In1/1 -> Memory/1, FixPt Relational Operator/1

== system CoCoSTLib_R2015b/Operators/Operators_LT/Always_LT /DetectIncrease ==
  note: Edge
  note: U(k)
  In1 : Inport
  FixPt Relational Operator : RelationalOperator  Operator=>  OutDataTypeStr=boolean  ZeroCross=off
  Memory : Memory
  Out1 : Outport
  wires:
  Memory/1 -> FixPt Relational Operator/2  "U(k-1)"
  In1/1 -> Memory/1, FixPt Relational Operator/1
  FixPt Relational Operator/1 -> Out1/1

== system CoCoSTLib_R2015b/Operators/Operators_LT/Always_LT_timewindows/DetectDecrease ==
  note: U(k)
  note: Edge
  In1 : Inport
  FixPt Relational Operator : RelationalOperator  Operator=<  OutDataTypeStr=boolean  ZeroCross=off
  Memory : Memory
  Out1 : Outport
  wires:
  FixPt Relational Operator/1 -> Out1/1
  In1/1 -> Memory/1, FixPt Relational Operator/1
  Memory/1 -> FixPt Relational Operator/2  "U(k-1)"

== system CoCoSTLib_R2015b/Operators/Operators_LT/Always_LT_timewindows/DetectIncrease ==
  note: U(k)
  note: Edge
  In1 : Inport
  FixPt Relational Operator : RelationalOperator  Operator=>  OutDataTypeStr=boolean  ZeroCross=off
  Memory : Memory
  Out1 : Outport
  wires:
  Memory/1 -> FixPt Relational Operator/2  "U(k-1)"
  In1/1 -> Memory/1, FixPt Relational Operator/1
  FixPt Relational Operator/1 -> Out1/1

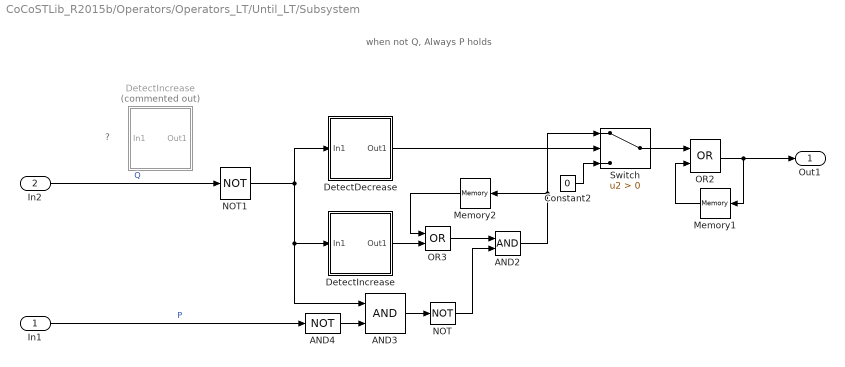
== system CoCoSTLib_R2015b/Operators/Operators_LT/Until_LT/Subsystem ==
  note: ?
  note: when not Q, Always P holds
  In1 : Inport
  In2 : Inport  Port=2
  AND2 : Logic  AllPortsSameDT=off  OutDataTypeStr=boolean
  AND3 : Logic  AllPortsSameDT=off  OutDataTypeStr=boolean
  AND4 : Logic  Operator=NOT  AllPortsSameDT=off  OutDataTypeStr=boolean
  Constant2 : Constant  Value=0  OutDataTypeStr=boolean
  DetectDecrease : Subsystem
  DetectIncrease : Subsystem  Commented=on
  "DetectIncrease " : Subsystem
  Memory1 : Memory
  Memory2 : Memory
  NOT : Logic  Operator=NOT  AllPortsSameDT=off  OutDataTypeStr=boolean
  NOT1 : Logic  Operator=NOT  IconShape=distinctive  AllPortsSameDT=off  OutDataTypeStr=boolean
  OR2 : Logic  Operator=OR  AllPortsSameDT=off  OutDataTypeStr=boolean
  OR3 : Logic  Operator=OR  AllPortsSameDT=off  OutDataTypeStr=boolean
  Switch : Switch  Criteria=u2 > Threshold
  Out1 : Outport
  wires:
  DetectDecrease/1(Out1) -> Switch/2
  Constant2/1 -> Switch/3
  OR3/1 -> AND2/1
  AND3/1 -> NOT/1
  AND4/1 -> AND3/2
  NOT1/1 -> DetectDecrease/1(In1), "DetectIncrease "/1(In1), AND3/1
  In1/1 -> AND4/1  "P"
  AND2/1 -> Memory2/1, Switch/1
  Memory2/1 -> OR3/1
  OR2/1 -> Out1/1, Memory1/1
  Memory1/1 -> OR2/2
  NOT/1 -> AND2/2
  "DetectIncrease "/1(Out1) -> OR3/2
  In2/1 -> NOT1/1  "Q"
  Switch/1 -> OR2/1

== system CoCoSTLib_R2015b/Operators/Operators_LT/Until_LT/Subsystem/DetectDecrease ==
  note: Edge
  note: U(k)
  In1 : Inport
  FixPt Relational Operator : RelationalOperator  Operator=<  OutDataTypeStr=boolean  ZeroCross=off
  Memory : Memory
  Out1 : Outport
  wires:
  Memory/1 -> FixPt Relational Operator/2  "U(k-1)"
  In1/1 -> FixPt Relational Operator/1, Memory/1
  FixPt Relational Operator/1 -> Out1/1

== system CoCoSTLib_R2015b/Operators/Operators_LT/Until_LT/Subsystem/DetectIncrease ==
  note: U(k)
  note: Edge
  In1 : Inport
  FixPt Relational Operator : RelationalOperator  Operator=>  OutDataTypeStr=boolean  ZeroCross=off
  Memory1 : Memory
  Out1 : Outport
  wires:
  Memory1/1 -> FixPt Relational Operator/2  "U(k-1)"
  In1/1 -> Memory1/1, FixPt Relational Operator/1
  FixPt Relational Operator/1 -> Out1/1

== system CoCoSTLib_R2015b/Operators/Operators_LT/Until_LT/Subsystem/DetectIncrease  ==
  note: Edge
  note: U(k)
  In1 : Inport
  FixPt Relational Operator : RelationalOperator  Operator=>  OutDataTypeStr=boolean  ZeroCross=off
  Memory : Memory
  Out1 : Outport
  wires:
  Memory/1 -> FixPt Relational Operator/2  "U(k-1)"
  In1/1 -> FixPt Relational Operator/1, Memory/1
  FixPt Relational Operator/1 -> Out1/1
